simulink model "FOC_physical_2"  (R2024b)
settings: Solver=FixedStepAuto  StartTime=0.0  StopTime=1  FixedStep=1e-6  RelTol=1e-3
undefined symbols (not defined in the file): alpha, DiscIntNeverNeededParam, Down, dspblkCoreblockFVToolHelper, gcbh, GPTRIP1SEL, Ki_current, Ki_q, Ki_s, Ki_speed, Kp_current, Kp_q, Kp_s, Kp_speed, lambda, lamdaM, Ld, Ls, ma, P, Rs, T_max, T_period, TZ1, Up, Vdc
libraries: c2802xlib x7, simulink x7, spsIGBTDiodeLib x6, spsCurrentMeasurementLib x3, eeStairGenerator x2, spsDCVoltageSourceLib x1, spsPermanentMagnetSynchronousMachineLib x1, mcbpositiondecoderlib x1, c281xlib x1, c280xlib x1, spspowerguiLib x1
(part 1 of 2)
settings Model: ExtModeTrigDuration=8  Creator=ahmed  LastModifiedBy=ahmed
settings SolverCC: ZeroCrossAlgorithm=Adaptive
settings OptimizationCC: DefaultParameterBehavior=Inlined  DefaultUnderspecifiedDataType=single  EnhancedBackFolding=on  PassReuseOutputArgsAs=Individual arguments  MaxStackSize=1024  OptimizeBlockOrder=speed  DifferentSizesBufferReuse=on  OptimizationCustomize=off  EfficientTunableParamExpr=on
settings DebuggingCC: IgnoredZcDiagnostic=none  ParameterTunabilityLossMsg=error
settings HardwareCC: ProdBitPerChar=16  ProdBitPerInt=16  ProdBitPerPointer=32  ProdBitPerSizeT=32  ProdBitPerPtrDiffT=32  ProdLargestAtomicInteger=Integer  ProdLargestAtomicFloat=None  ProdWordSize=16  ProdLongLongMode=on  ProdHWDeviceType=Texas Instruments->C2000  HardwareBoardFeatureSet=SoCBlockset
settings SFSimCC: MATLABDynamicMemAlloc=off
settings RTWCC: Description=Embedded Coder  SystemTargetFile=ert.tlc  HardwareBoard=TI Delfino F28379D LaunchPad  TemplateMakefile=ert_default_tmf  Toolchain=Texas Instruments Code Composer Studio (C2000)  CodeProfilingSaveOptions=MetricsOnly
settings CodeAppCC: ForceParamTrailComments=on  IgnoreCustomStorageClasses=off  OperatorAnnotations=on  SimulinkDataObjDesc=on  SFDataObjDesc=on  InsertBlockDesc=on
settings ERTTargetCC: CodeReplacementLibrary=TI C28x  ExtModeTransport=4  ExtModeStaticAlloc=on  ExtModeAutomaticAllocSize=off  ExtModeStaticAllocSize=10000  ExtModeMexFile=ext_xcp  ExtModeIntrfLevel=Level2 - Open

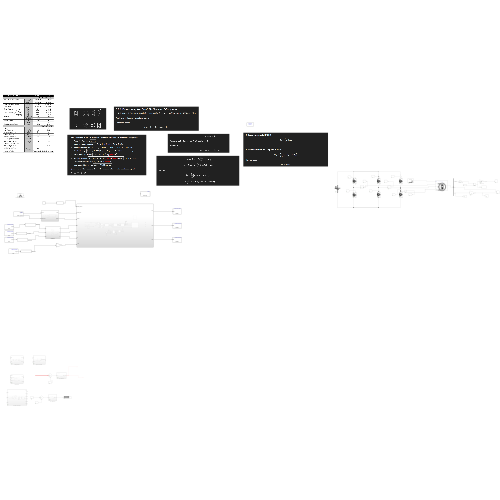
[thumbnail: Simulink's stored preview of the top-level diagram]
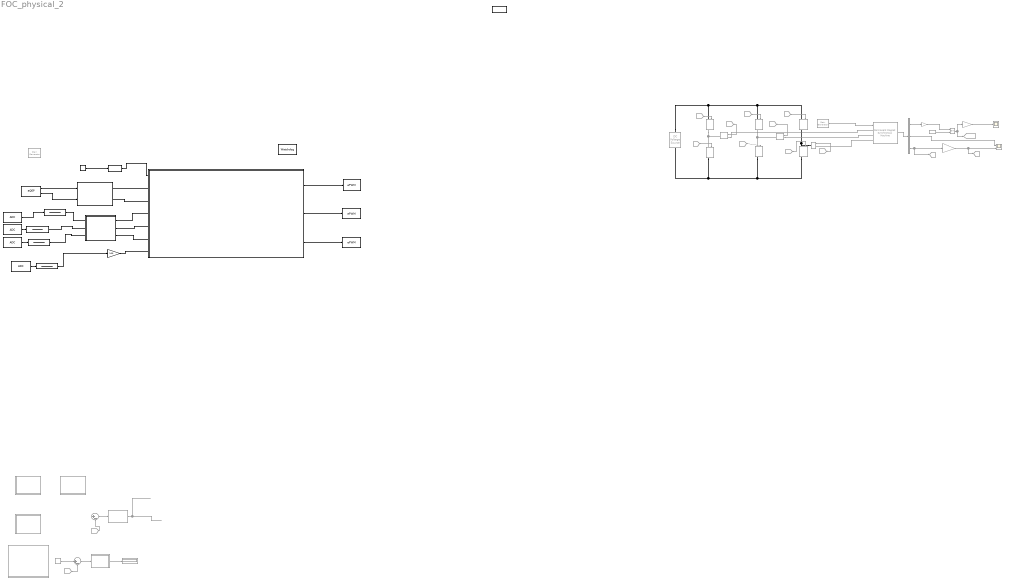
== system FOC_physical_2 ==
  0 to 2pi : Math  Commented=on  Operator=rem
  ADC : c2802xlib/ADC  blkParamProc=C2000_Type4  ADCModule=A  samplingMode=Single sample mode  ADCResolution=12-bit (Single-ended input)  useSOC1=SOC0  useSOC2=SOC0_SOC1  SOCAcquisitionWindow=15  SOCTriggerSource=Software  SOCInterruptTrigger=No ADCINT  Ts=50e-6  dType=uint16  postInterrupt=off  interruptSel=ADCINT1  ADCINTContinuous=on  endma=off  chdma=1  conv1=ADCINA0  conv2=ADCINA0 and ADCINB0  conv1_Type4=ADCIN0  conv2_Type4=ADCIN0 and ADCIN1
      settings: LibrarySourceBlock=c2837xDlib/ADC
  ADC1 : c2802xlib/ADC  blkParamProc=C2000_Type4  ADCModule=A  samplingMode=Single sample mode  ADCResolution=12-bit (Single-ended input)  useSOC1=SOC1  useSOC2=SOC0_SOC1  SOCAcquisitionWindow=15  SOCTriggerSource=ePWM1_ADCSOCA  SOCInterruptTrigger=No ADCINT  Ts=1e-6  dType=uint16  postInterrupt=off  interruptSel=ADCINT1  ADCINTContinuous=on  endma=off  chdma=1  conv1=ADCINA0  conv2=ADCINA0 and ADCINB0  conv1_Type4=ADCIN1  conv2_Type4=ADCIN0 and ADCIN1
      settings: LibrarySourceBlock=c2837xDlib/ADC
  ADC2 : c2802xlib/ADC  blkParamProc=C2000_Type4  ADCModule=A  samplingMode=Single sample mode  ADCResolution=12-bit (Single-ended input)  useSOC1=SOC2  useSOC2=SOC0_SOC1  SOCAcquisitionWindow=15  SOCTriggerSource=ePWM1_ADCSOCA  SOCInterruptTrigger=No ADCINT  Ts=1e-6  dType=uint16  postInterrupt=off  interruptSel=ADCINT1  ADCINTContinuous=on  endma=off  chdma=1  conv1=ADCINA0  conv2=ADCINA0 and ADCINB0  conv1_Type4=ADCIN2  conv2_Type4=ADCIN0 and ADCIN1
      settings: LibrarySourceBlock=c2837xDlib/ADC
  ADC3 : c2802xlib/ADC  blkParamProc=C2000_Type4  ADCModule=A  samplingMode=Single sample mode  ADCResolution=12-bit (Single-ended input)  useSOC1=SOC3  useSOC2=SOC0_SOC1  SOCAcquisitionWindow=15  SOCTriggerSource=ePWM1_ADCSOCA  SOCInterruptTrigger=No ADCINT  Ts=1e-6  dType=uint16  postInterrupt=off  interruptSel=ADCINT1  ADCINTContinuous=on  endma=off  chdma=1  conv1=ADCINA0  conv2=ADCINA0 and ADCINB0  conv1_Type4=ADCIN3  conv2_Type4=ADCIN0 and ADCIN1
      settings: LibrarySourceBlock=c2837xDlib/ADC
  Bus Selector : BusSelector  Commented=on  OutputSignals=theta,Te,w
  "Calibration " : Subsystem
  Cast To Double : DataTypeConversion  OutDataTypeStr=double  SaturateOnIntegerOverflow=off  RndMeth=Floor
  Constant : Constant  Value=1500  OutDataTypeStr=double
  Constant4 : Constant  Commented=on  Value=2*pi
  Current Measurement : spsCurrentMeasurementLib/Current Measurement  Commented=on  PhasorSimulation=off  OutputType=Complex  PSBequivalent=0
  Current Measurement1 : spsCurrentMeasurementLib/Current Measurement  Commented=on  PhasorSimulation=off  OutputType=Complex  PSBequivalent=0
  Current Measurement2 : spsCurrentMeasurementLib/Current Measurement  Commented=on  PhasorSimulation=off  OutputType=Complex  PSBequivalent=0
  DC Voltage Source : spsDCVoltageSourceLib/DC Voltage Source  Commented=on  Amplitude=Vdc  Measurements=None
  "Decoupling " : Subsystem  Commented=on
  Discrete Transfer Fcn{1..3,8} (4 alike) : DiscreteTransferFcn  LoadFcn=dspblkCoreblockFVToolHelper(gcbh,'load');  Numerator=[alpha]  Denominator=[1 (alpha)-1]  RndMeth=Nearest
      settings: CopyFcn=dspblkCoreblockFVToolHelper(gcbh,'copy');  DeleteFcn=dspblkCoreblockFVToolHelper(gcbh,'close');  ModelCloseFcn=dspblkCoreblockFVToolHelper(gcbh,'close');  PreSaveFcn=dspblkCoreblockFVToolHelper(gcbh,'presave');  PostSaveFcn=dspblkCoreblockFVToolHelper(gcbh,'postsave');  CloseFcn=dspblkCoreblockFVToolHelper(gcbh,'close');
  Display5 : Display  Commented=on
  From13 : From  Commented=on  GotoTag=Iq  TagVisibility=global
  From14 : From  Commented=on  GotoTag=Id  TagVisibility=global
  From2 : From  Commented=on  GotoTag=S1  TagVisibility=global
  From3 : From  Commented=on  GotoTag=S3  TagVisibility=global
  From4 : From  Commented=on  GotoTag=S5  TagVisibility=global
  From5 : From  Commented=on  GotoTag=S4  TagVisibility=global
  From6 : From  Commented=on  GotoTag=S6  TagVisibility=global
  From7 : From  Commented=on  GotoTag=S2  TagVisibility=global
  Gain : Gain  Commented=on  Gain=60/(2*pi)
  Gain1 : Gain  Gain=100
  Goto : Goto  Commented=on  GotoTag=N_act
  Goto1 : Goto  Commented=on  GotoTag=theta_rad  TagVisibility=global
  Goto12 : Goto  Commented=on  GotoTag=Ia
  Goto13 : Goto  Commented=on  GotoTag=Ib
  Goto14 : Goto  Commented=on  GotoTag=Ic
  Goto8 : Goto  Commented=on  GotoTag=W_act
  IGBT/Diode{,1..5} (6 alike) : spsIGBTDiodeLib/IGBT//Diode  Commented=on  Ron=1e-3  Rs=1e5  Cs=inf  Measurements=on
  Id : Constant  Commented=on  Value=0
  PI_controller : Subsystem  Commented=on
  PI_controller1 : Subsystem  Commented=on
  Permanent Magnet Synchronous Machine : spsPermanentMagnetSynchronousMachineLib/Permanent Magnet Synchronous Machine  Commented=on  NbPhases=3  FluxDistribution=Sinusoidal  RotorType=Round  MechanicalLoad=Torque Tm  PresetModel=No  ShowDetailedParameters=on  MeasurementBus=on  Resistance=Rs  Inductance=8.5e-3  dqInductances=[6.2e-3 6.2e-3]  La=Ls  MachineConstant=Flux linkage established by magnets (V.s)  Flux=.0620  VoltageCst=44.9822  TorqueCst=0.372  Flat=120  Mechanical=[2.6e-5 9.55e-5 4 .03]  PolePairs=4  InitialConditions=[0,0, 0,0]  InitialConditions5ph=[0 0 0 0 0 0]  RefAngle=Aligned with phase A axis (original Park)  IterativeDiscreteModel=Trapezoidal non iterative  TsBlock=-1  TsPowergui=0
  SPEED_TEST_VALUES : eeStairGenerator/Stair Generator  Commented=on  LabelModeActiveChoice=Discrete  TimeInput=[0.2 .6 1 1.3 1.8 2.2 3]  AmplitudeInput=[200 300 1000 4000 4500 2000 0]  SampleTime=1e-5  RepeatPattern=off
      settings: LibrarySourceBlock=ee_sl_lib/General Control/Stair Generator
  SVPWM Technique : Subsystem  Commented=on
  Scope : Scope  Commented=on
  Scope1 : Scope  Commented=on  NumInputPorts=2
  "Speed Controller " : Subsystem  Commented=on
  Stair Generator2 : eeStairGenerator/Stair Generator  Commented=on  LabelModeActiveChoice=Discrete  TimeInput=[0.3 .7]  AmplitudeInput=[.6 1]  SampleTime=1e-5  RepeatPattern=off  OutDataTypeStr=double
      settings: LibrarySourceBlock=ee_sl_lib/General Control/Stair Generator
  Subsystem : Subsystem
  Subsystem1 : Subsystem
  Sum1 : Sum  Commented=on  Inputs=|+-
  Sum2 : Sum  Commented=on  Inputs=|+-
  Voltage limits : Subsystem  Commented=on
  Watchdog : c281xlib/Watchdog  resetsrc=Input port  sample=-1
      settings: LibrarySourceBlock=c2837xDlib/Watchdog
  ePWM11 : c2802xlib/ePWM  PwmType=C2000_Type4  useModule=ePWM1  ePWMxLINKTBPRD=Not Linked  periodUnits=Clock cycles  timerSource=Specify via dialog  timerPeriod_clk=10000  timerPeriod_sec=0.0001  tbshadow=Counter equals to zero  countingMode=Up-Down  phaseActiveEnable=Disable  phaseDirection=Count down after sync  phaseActive=0  synchronizationEnable=off  dcaevt1Sync=off  dcbevt1Sync=off  synchronizationOption=Counter equals to zero (CTR=Zero)  dcbevt1SyncOut=off  dcaevt1SyncOut=off  cmpdSyncOut=off  cmpcSyncOut=off  cmpbSyncOut=off  zeroSyncOut=off  swfSyncOut=off  perSynchronizationOption=Counter equals to period (CTR=PRD)  clockPrescale=1  HSclockPrescale=1  enswap=off  ePWMxAStatus=on  ePWMxAactionLogic1=Do nothing  ePWMxAactionLogic2=Do nothing  ePWMxAactionLogic3=Clear  ePWMxAactionLogic4=Set  ePWMxAactionLogic5=Do nothing  ePWMxAactionLogic6=Do nothing  ePWMxACSFenable=off  ePWMxACSFvalue=Forcing disable  ePWMxASFreload=Zero  ePWMxBStatus=on  ePWMxBactionLogic1=Do nothing  ePWMxBactionLogic2=Do nothing  ePWMxBactionLogic3=Set  ePWMxBactionLogic4=Clear  ePWMxBactionLogic5=Do nothing  ePWMxBactionLogic6=Do nothing  ePWMxBCSFenable=off  ePWMxBCSFvalue=Forcing disable  ePWMxBSFreload=Zero  ePWNxBOutWay=off  ePWMxLINKCMPA=Not Linked  CMPAUnits=Clock cycles  CMPASource=Input port  CMPAValue_per=0  CMPAValue_clk=0  enCMPAshadow=Counter equals to zero (CTR=Zero)  ePWMxLINKCMPB=Not Linked  CMPBUnits=Clock cycles  CMPBSource=Specify via dialog  CMPBValue_per=50  CMPBValue_clk=32000  enCMPBshadow=Counter equals to zero (CTR=Zero)  ePWMxLINKCMPC=Not Linked  CMPCUnits=Clock cycles  CMPCSource=Specify via dialog  CMPCValue_per=50  CMPCValue_clk=32000  enCMPCshadow=Counter equals to zero (CTR=Zero)  ePWMxLINKCMPD=Not Linked  CMPDUnits=Clock cycles  CMPDSource=Specify via dialog  CMPDValue_per=50  CMPDValue_clk=32000  enCMPDshadow=Counter equals to zero (CTR=Zero)  enableDBePWMxA=on  enableDBePWMxB=on  enhalfcycle=off  DBpolarity=Active high complementary (AHC)  DBedgeDelay=Positive  DBSource_ePWMxA=ePWMxA  DBSource_ePWMxB=ePWMxA  DBPeriodUnits=Clock cycles  DBperiodSource=Specify via dialog  REDperiod=400  FEDperiod=400  REDperiod_sec=0  FEDperiod_sec=0  LoadModeDBRED=Immediate without using shadow  LoadModeDBFED=Immediate without using shadow  adcstartModuleA=on  adcrequestEventA=First event  adcstartEventA=Digital Compare Module A Event 1 start of conversion (DCAEVT1.soc)  adcstartEventA_type2=Counter equals to period (CTR=PRD)  adcstartModuleB=off  adcrequestEventB=First event  adcstartEventB=Counter equals to zero (CTR=Zero)  adcstartEventB_type2=Counter equals to zero (CTR=Zero)  intEn=on  intPrd=First event  intSel=Counter equals to zero (CTR=Zero)  intSel_type2=Counter equals to period (CTR=PRD)  hrpe=off  enHRPWM=off  HRPWM_LoadMode=Counter equals to period (CTR=PRD)  HRPWM_CTLMode=Duty or Period control mode  HRPWM_EDGMode=Both edge  hrpeb=off  enHRPWMB=off  HRPWM_LoadModeB=Counter equals to zero (CTR=ZERO)  HRPWM_CTLModeB=Duty or Period control mode  HRPWM_EDGModeB=Both edge  enHRDBRED=off  enHRDBFED=off  enSFO=on  enautoconv=on  chopperEnable=off  chopperFrequency=1  chopperFirstwidth=1  chopperDuty=12.5%  tripZonesource=Specify via dialog  tzselOSHT1=off  tzselOSHT2=off  tzselOSHT3=off  tzselOSHT4=off  tzselOSHT5=off  tzselOSHT6=off  tzselOSHDCAEV1=off  tzselOSHDCBEV1=off  tzselCBC1=off  tzselCBC2=off  tzselCBC3=off  tzselCBC4=off  tzselCBC5=off  tzselCBC6=off  tzselCBCDCAEV2=off  tzselCBCDCBEV2=off  enTzOstIntr=off  enTzCbcIntr=off  enTzDCAEVT1Intr=off  enTzDCAEVT2Intr=off  enTzDCBEVT1Intr=off  enTzDCBEVT2Intr=off  tzclrCBCLatch=Counter equals to zero (CTR=Zero)  ePWMxAforced=No action  ePWMxBforced=No action  DCAEVT1forced=No action  DCBEVT1forced=No action  DCAEVT2forced=No action  DCBEVT2forced=No action  dcah=Trip Zone 1 input (TZ1)  dcal=Trip Zone 2 input (TZ2)  dcbh=Trip Zone 1 input (TZ1)  dcbl=Trip Zone 2 input (TZ2)  dcah_type2=GPTRIP1SEL/(TZ1)  dcal_type2=GPTRIP1SEL/(TZ1)  dcbh_type2=GPTRIP1SEL/(TZ1)  dcbl_type2=GPTRIP1SEL/(TZ1)  gendcaevt1=Event disabled  gendcaevt2=Event disabled  gendcbevt1=Event disabled  gendcbevt2=Event disabled  dcaevt1src=DCAEVT1 with sync  dcaevt2src=DCAEVT2 with sync  dcbevt1src=DCBEVT1 with sync  dcbevt2src=DCBEVT2 with sync  pulsesel=Counter equals to zero (CTR=Zero)  blankinv=off  blankoffset=0  blankwidth=0  evsrcsel=Filtered version of DCAEVT1 (DCAEVT1FILT)  encape=off
      settings: LibrarySourceBlock=c2837xDlib/ePWM
  ePWM12 : c2802xlib/ePWM  PwmType=C2000_Type4  useModule=ePWM2  ePWMxLINKTBPRD=Not Linked  periodUnits=Clock cycles  timerSource=Specify via dialog  timerPeriod_clk=10000  timerPeriod_sec=0.0001  tbshadow=Counter equals to zero  countingMode=Up-Down  phaseActiveEnable=Disable  phaseDirection=Count down after sync  phaseActive=0  synchronizationEnable=off  dcaevt1Sync=off  dcbevt1Sync=off  synchronizationOption=Disable  dcbevt1SyncOut=off  dcaevt1SyncOut=off  cmpdSyncOut=off  cmpcSyncOut=off  cmpbSyncOut=off  zeroSyncOut=off  swfSyncOut=off  perSynchronizationOption=Counter equals to period (CTR=PRD)  clockPrescale=1  HSclockPrescale=1  enswap=off  ePWMxAStatus=on  ePWMxAactionLogic1=Do nothing  ePWMxAactionLogic2=Do nothing  ePWMxAactionLogic3=Clear  ePWMxAactionLogic4=Set  ePWMxAactionLogic5=Do nothing  ePWMxAactionLogic6=Do nothing  ePWMxACSFenable=off  ePWMxACSFvalue=Forcing disable  ePWMxASFreload=Zero  ePWMxBStatus=on  ePWMxBactionLogic1=Do nothing  ePWMxBactionLogic2=Do nothing  ePWMxBactionLogic3=Set  ePWMxBactionLogic4=Clear  ePWMxBactionLogic5=Do nothing  ePWMxBactionLogic6=Do nothing  ePWMxBCSFenable=off  ePWMxBCSFvalue=Forcing disable  ePWMxBSFreload=Zero  ePWNxBOutWay=off  ePWMxLINKCMPA=Not Linked  CMPAUnits=Clock cycles  CMPASource=Input port  CMPAValue_per=0  CMPAValue_clk=0  enCMPAshadow=Counter equals to zero (CTR=Zero)  ePWMxLINKCMPB=Not Linked  CMPBUnits=Clock cycles  CMPBSource=Specify via dialog  CMPBValue_per=50  CMPBValue_clk=32000  enCMPBshadow=Counter equals to zero (CTR=Zero)  ePWMxLINKCMPC=Not Linked  CMPCUnits=Clock cycles  CMPCSource=Specify via dialog  CMPCValue_per=50  CMPCValue_clk=32000  enCMPCshadow=Counter equals to zero (CTR=Zero)  ePWMxLINKCMPD=Not Linked  CMPDUnits=Clock cycles  CMPDSource=Specify via dialog  CMPDValue_per=50  CMPDValue_clk=32000  enCMPDshadow=Counter equals to zero (CTR=Zero)  enableDBePWMxA=on  enableDBePWMxB=on  enhalfcycle=off  DBpolarity=Active high complementary (AHC)  DBedgeDelay=Positive  DBSource_ePWMxA=ePWMxA  DBSource_ePWMxB=ePWMxA  DBPeriodUnits=Clock cycles  DBperiodSource=Specify via dialog  REDperiod=400  FEDperiod=400  REDperiod_sec=0  FEDperiod_sec=0  LoadModeDBRED=Immediate without using shadow  LoadModeDBFED=Immediate without using shadow  adcstartModuleA=on  adcrequestEventA=First event  adcstartEventA=Digital Compare Module A Event 1 start of conversion (DCAEVT1.soc)  adcstartEventA_type2=Counter equals to period (CTR=PRD)  adcstartModuleB=off  adcrequestEventB=First event  adcstartEventB=Counter equals to zero (CTR=Zero)  adcstartEventB_type2=Counter equals to zero (CTR=Zero)  intEn=on  intPrd=First event  intSel=Counter equals to zero (CTR=Zero)  intSel_type2=Counter equals to period (CTR=PRD)  hrpe=off  enHRPWM=off  HRPWM_LoadMode=Counter equals to period (CTR=PRD)  HRPWM_CTLMode=Duty or Period control mode  HRPWM_EDGMode=Both edge  hrpeb=off  enHRPWMB=off  HRPWM_LoadModeB=Counter equals to zero (CTR=ZERO)  HRPWM_CTLModeB=Duty or Period control mode  HRPWM_EDGModeB=Both edge  enHRDBRED=off  enHRDBFED=off  enSFO=on  enautoconv=on  chopperEnable=off  chopperFrequency=1  chopperFirstwidth=1  chopperDuty=12.5%  tripZonesource=Specify via dialog  tzselOSHT1=off  tzselOSHT2=off  tzselOSHT3=off  tzselOSHT4=off  tzselOSHT5=off  tzselOSHT6=off  tzselOSHDCAEV1=off  tzselOSHDCBEV1=off  tzselCBC1=off  tzselCBC2=off  tzselCBC3=off  tzselCBC4=off  tzselCBC5=off  tzselCBC6=off  tzselCBCDCAEV2=off  tzselCBCDCBEV2=off  enTzOstIntr=off  enTzCbcIntr=off  enTzDCAEVT1Intr=off  enTzDCAEVT2Intr=off  enTzDCBEVT1Intr=off  enTzDCBEVT2Intr=off  tzclrCBCLatch=Counter equals to zero (CTR=Zero)  ePWMxAforced=No action  ePWMxBforced=No action  DCAEVT1forced=No action  DCBEVT1forced=No action  DCAEVT2forced=No action  DCBEVT2forced=No action  dcah=Trip Zone 1 input (TZ1)  dcal=Trip Zone 2 input (TZ2)  dcbh=Trip Zone 1 input (TZ1)  dcbl=Trip Zone 2 input (TZ2)  dcah_type2=GPTRIP1SEL/(TZ1)  dcal_type2=GPTRIP1SEL/(TZ1)  dcbh_type2=GPTRIP1SEL/(TZ1)  dcbl_type2=GPTRIP1SEL/(TZ1)  gendcaevt1=Event disabled  gendcaevt2=Event disabled  gendcbevt1=Event disabled  gendcbevt2=Event disabled  dcaevt1src=DCAEVT1 with sync  dcaevt2src=DCAEVT2 with sync  dcbevt1src=DCBEVT1 with sync  dcbevt2src=DCBEVT2 with sync  pulsesel=Counter equals to zero (CTR=Zero)  blankinv=off  blankoffset=0  blankwidth=0  evsrcsel=Filtered version of DCAEVT1 (DCAEVT1FILT)  encape=off
      settings: LibrarySourceBlock=c2837xDlib/ePWM
  ePWM13 : c2802xlib/ePWM  PwmType=C2000_Type4  useModule=ePWM4  ePWMxLINKTBPRD=Not Linked  periodUnits=Clock cycles  timerSource=Specify via dialog  timerPeriod_clk=10000  timerPeriod_sec=0.0001  tbshadow=Counter equals to zero  countingMode=Up-Down  phaseActiveEnable=Disable  phaseDirection=Count down after sync  phaseActive=0  synchronizationEnable=off  dcaevt1Sync=off  dcbevt1Sync=off  synchronizationOption=Disable  dcbevt1SyncOut=off  dcaevt1SyncOut=off  cmpdSyncOut=off  cmpcSyncOut=off  cmpbSyncOut=off  zeroSyncOut=off  swfSyncOut=off  perSynchronizationOption=Counter equals to period (CTR=PRD)  clockPrescale=1  HSclockPrescale=1  enswap=off  ePWMxAStatus=on  ePWMxAactionLogic1=Do nothing  ePWMxAactionLogic2=Do nothing  ePWMxAactionLogic3=Clear  ePWMxAactionLogic4=Set  ePWMxAactionLogic5=Do nothing  ePWMxAactionLogic6=Do nothing  ePWMxACSFenable=off  ePWMxACSFvalue=Forcing disable  ePWMxASFreload=Zero  ePWMxBStatus=on  ePWMxBactionLogic1=Do nothing  ePWMxBactionLogic2=Do nothing  ePWMxBactionLogic3=Set  ePWMxBactionLogic4=Clear  ePWMxBactionLogic5=Do nothing  ePWMxBactionLogic6=Do nothing  ePWMxBCSFenable=off  ePWMxBCSFvalue=Forcing disable  ePWMxBSFreload=Zero  ePWNxBOutWay=off  ePWMxLINKCMPA=Not Linked  CMPAUnits=Clock cycles  CMPASource=Input port  CMPAValue_per=0  CMPAValue_clk=0  enCMPAshadow=Counter equals to zero (CTR=Zero)  ePWMxLINKCMPB=Not Linked  CMPBUnits=Clock cycles  CMPBSource=Specify via dialog  CMPBValue_per=50  CMPBValue_clk=32000  enCMPBshadow=Counter equals to zero (CTR=Zero)  ePWMxLINKCMPC=Not Linked  CMPCUnits=Clock cycles  CMPCSource=Specify via dialog  CMPCValue_per=50  CMPCValue_clk=32000  enCMPCshadow=Counter equals to zero (CTR=Zero)  ePWMxLINKCMPD=Not Linked  CMPDUnits=Clock cycles  CMPDSource=Specify via dialog  CMPDValue_per=50  CMPDValue_clk=32000  enCMPDshadow=Counter equals to zero (CTR=Zero)  enableDBePWMxA=on  enableDBePWMxB=on  enhalfcycle=off  DBpolarity=Active high complementary (AHC)  DBedgeDelay=Positive  DBSource_ePWMxA=ePWMxA  DBSource_ePWMxB=ePWMxA  DBPeriodUnits=Clock cycles  DBperiodSource=Specify via dialog  REDperiod=400  FEDperiod=400  REDperiod_sec=0  FEDperiod_sec=0  LoadModeDBRED=Immediate without using shadow  LoadModeDBFED=Immediate without using shadow  adcstartModuleA=on  adcrequestEventA=First event  adcstartEventA=Digital Compare Module A Event 1 start of conversion (DCAEVT1.soc)  adcstartEventA_type2=Counter equals to period (CTR=PRD)  adcstartModuleB=off  adcrequestEventB=First event  adcstartEventB=Counter equals to zero (CTR=Zero)  adcstartEventB_type2=Counter equals to zero (CTR=Zero)  intEn=on  intPrd=First event  intSel=Counter equals to zero (CTR=Zero)  intSel_type2=Counter equals to period (CTR=PRD)  hrpe=off  enHRPWM=off  HRPWM_LoadMode=Counter equals to period (CTR=PRD)  HRPWM_CTLMode=Duty or Period control mode  HRPWM_EDGMode=Both edge  hrpeb=off  enHRPWMB=off  HRPWM_LoadModeB=Counter equals to zero (CTR=ZERO)  HRPWM_CTLModeB=Duty or Period control mode  HRPWM_EDGModeB=Both edge  enHRDBRED=off  enHRDBFED=off  enSFO=on  enautoconv=on  chopperEnable=off  chopperFrequency=1  chopperFirstwidth=1  chopperDuty=12.5%  tripZonesource=Specify via dialog  tzselOSHT1=off  tzselOSHT2=off  tzselOSHT3=off  tzselOSHT4=off  tzselOSHT5=off  tzselOSHT6=off  tzselOSHDCAEV1=off  tzselOSHDCBEV1=off  tzselCBC1=off  tzselCBC2=off  tzselCBC3=off  tzselCBC4=off  tzselCBC5=off  tzselCBC6=off  tzselCBCDCAEV2=off  tzselCBCDCBEV2=off  enTzOstIntr=off  enTzCbcIntr=off  enTzDCAEVT1Intr=off  enTzDCAEVT2Intr=off  enTzDCBEVT1Intr=off  enTzDCBEVT2Intr=off  tzclrCBCLatch=Counter equals to zero (CTR=Zero)  ePWMxAforced=No action  ePWMxBforced=No action  DCAEVT1forced=No action  DCBEVT1forced=No action  DCAEVT2forced=No action  DCBEVT2forced=No action  dcah=Trip Zone 1 input (TZ1)  dcal=Trip Zone 2 input (TZ2)  dcbh=Trip Zone 1 input (TZ1)  dcbl=Trip Zone 2 input (TZ2)  dcah_type2=GPTRIP1SEL/(TZ1)  dcal_type2=GPTRIP1SEL/(TZ1)  dcbh_type2=GPTRIP1SEL/(TZ1)  dcbl_type2=GPTRIP1SEL/(TZ1)  gendcaevt1=Event disabled  gendcaevt2=Event disabled  gendcbevt1=Event disabled  gendcbevt2=Event disabled  dcaevt1src=DCAEVT1 with sync  dcaevt2src=DCAEVT2 with sync  dcbevt1src=DCBEVT1 with sync  dcbevt2src=DCBEVT2 with sync  pulsesel=Counter equals to zero (CTR=Zero)  blankinv=off  blankoffset=0  blankwidth=0  evsrcsel=Filtered version of DCAEVT1 (DCAEVT1FILT)  encape=off
      settings: LibrarySourceBlock=c2837xDlib/ePWM
  eQEP : c280xlib/eQEP  useModule=eQEP1  pcInputmode=Quadrature-count  externalClockrate=2x resolution: Count the rising/falling edge  swapPolarityselection=Clockwise  qdfOutputport=off  qapPolarityselection=off  qbpPolarityselection=off  qipPolarityselection=off  qspPolarityselection=off  igatePolarityselection=off  sampleTime=0.0001  pcOutputport=on  pcMaximumvalue=4*2000  indexInitializationcheck=off  indexInitializationevent=Rising edge  strobeInitializationcheck=off  strobeInitializationevent=Rising edge  softwareInitializationcheck=off  softwareInitializationsource=Set to init value at start up  softwareInitializationmode=on  pcInitialvalue=2147483648  pcResetmode=Reset on the maximum position  ieloutputport=on  indexEventlatch=Rising edge  seloutputport=off  strobeEventlatch=Rising edge  pcefOutputport=off  enableEqepcapture=on  qctmrOutputport=off  qcprdOutputport=off  captureTimerprescaler=128  upEventprescaler=128  overflowErrorflag=off  directionErrorflag=off  captureTimerposition=On position counter read  unitTimerperiod=100000000  captureTimerlatch=off  capturePeriodlatch=off  positionCounterlatch=off  soenPolarityselection=off  spselPolarityselection=Index pin is used for sync output  compareValuesource=Specify via dialog  shadowMode=Load on QPOSCNT=0  compareValue=4294967295  syncOutputwidth=1  polaritySyncoutput=Active high  watchdogEnable=off  watchdogTimer=65535  outport1Datatype=auto  outport2Datatype=auto  outport3Datatype=auto  outport4Datatype=auto  outport5Datatype=auto  outport6Datatype=auto  outport7Datatype=auto  outport8Datatype=auto  outport9Datatype=auto  outport10Datatype=auto  outport11Datatype=auto  outport12Datatype=auto  eqepinterrupt_pce=off  eqepinterrupt_qpe=off  eqepinterrupt_qdc=off  eqepinterrupt_wto=off  eqepinterrupt_pcu=off  eqepinterrupt_pco=off  eqepinterrupt_pcr=off  eqepinterrupt_pcm=off  eqepinterrupt_sel=off  eqepinterrupt_iel=off  eqepinterrupt_uto=off  pheOutputport=off  watchdogOutputport=off  outport13Datatype=auto  outport14Datatype=auto
      settings: LibrarySourceBlock=c2837xDlib/eQEP
  mech to elec : Gain  Commented=on  Gain=P
  powergui : spspowerguiLib/powergui  Priority=1  SimulationMode=Discrete  SampleTime=1e-5  frequency=60  Iterations=50  frequencyindice=0  Pbase=100e6  ErrMax=1e-4  UnitsV=kV  UnitsW=MW  buscounter=0  FunctionMessages=off  echomessages=off  EnableUseOfTLC=off  CurrentSourceSwitches=off  DisableSnubberDevices=off  DisableRonSwitches=off  DisableVfSwitches=off  DisplayEquations=off  AutomaticDiscreteSolvers=off  SolverType=Tustin/Backward Euler (TBE)  Interpol=off  ExternalGateDelay=off  methode=off  Ts=100  x0status=blocks  SPID=on  SwTol=0  HookPort=off  NonlinearTolerance=1e-4  nMaxIteration=100  ContinueOnMaxIteration=off  RestoreLinks=warning  ResistiveCurrentMeasurement=off  Frange=[0:2:500]  Ylog=off  Xlog=on  ShowGrid=off  save=off  variable=ZData  structure=0  ZoomFFT=off  StartTime=0.0  cycles=1  DisplayStyle=1  fundamental=60  FreqAxis=off  MaxFrequency=1000  frequencyindicesteady=1  RmsSteady=1  display=off
  rad to deg : Gain  Commented=on  Gain=180/pi
  wires:
  Permanent Magnet Synchronous Machine/1 -> Bus Selector/1
  From3/1 -> IGBT/Diode1/1
  From6/1 -> IGBT/Diode3/1
  From4/1 -> IGBT/Diode4/1
  From5/1 -> IGBT/Diode2/1
  From2/1 -> IGBT/Diode/1
  From7/1 -> IGBT/Diode5/1
  PI_controller1/1(Vd_hat) -> Display5/1
  Id/1 -> Sum1/1
  From14/1 -> Sum1/2
  Current Measurement/1 -> Goto12/1
  Current Measurement1/1 -> Goto13/1
  Sum1/1 -> PI_controller1/1(e_d)
  ? -> Sum2/1
  Sum2/1 -> PI_controller/1(e_q)
  PI_controller/1(Vq_hat) -> ?
  From13/1 -> Sum2/2
  Bus Selector/2 -> Scope1/1  "<Te>"
  Bus Selector/3 -> Goto8/1, Gain/1  "<w>"
  Bus Selector/1 -> mech to elec/1  "<theta>"
  0 to 2pi/1 -> rad to deg/1, Goto1/1
  Constant4/1 -> 0 to 2pi/2
  rad to deg/1 -> Scope/1  "degrees"
  mech to elec/1 -> 0 to 2pi/1
  Gain/1 -> Goto/1, Scope1/2
  Current Measurement2/1 -> Goto14/1
  Stair Generator2/1 -> Permanent Magnet Synchronous Machine/1
  Subsystem/1(TS1) -> ePWM11/1
  Subsystem/2(TS3) -> ePWM12/1
  Subsystem/3(TS5) -> ePWM13/1
  eQEP/1 -> Subsystem1/1(Count)
  eQEP/2 -> Subsystem1/2(IndexCount)
  Subsystem1/1(theta) -> Subsystem/2(Theata_elec)
  Subsystem1/2(Speed) -> Subsystem/3(Speed)
  ADC/1 -> Discrete Transfer Fcn8/1
  ADC1/1 -> Discrete Transfer Fcn1/1
  ADC2/1 -> Discrete Transfer Fcn2/1
  "Calibration "/1(Out1) -> Subsystem/4(Iu)
  "Calibration "/2(Out2) -> Subsystem/5(Iv)
  "Calibration "/3(Out3) -> Subsystem/6(Iw)
  ADC3/1 -> Discrete Transfer Fcn3/1
  Gain1/1 -> Subsystem/7(V_DC)
  Constant/1 -> Cast To Double/1
  Cast To Double/1 -> Subsystem/1(SPEED_INPUT)
  Discrete Transfer Fcn8/1 -> "Calibration "/1(In1)  "Discrete TF"
  Discrete Transfer Fcn1/1 -> "Calibration "/2(In2)  "Discrete TF"
  Discrete Transfer Fcn2/1 -> "Calibration "/3(In3)  "Discrete TF"
  Discrete Transfer Fcn3/1 -> Gain1/1  "Discrete TF"
  connections:
  DC Voltage Source/RConn1 -- IGBT/Diode4/LConn1 -- IGBT/Diode1/LConn1 -- IGBT/Diode/LConn1
  Current Measurement/LConn1 -- IGBT/Diode/RConn1 -- IGBT/Diode2/LConn1
  Current Measurement2/LConn1 -- IGBT/Diode4/RConn1 -- IGBT/Diode5/LConn1
  DC Voltage Source/LConn1 -- IGBT/Diode5/RConn1 -- IGBT/Diode3/RConn1 -- IGBT/Diode2/RConn1
  Current Measurement1/LConn1 -- IGBT/Diode1/RConn1 -- IGBT/Diode3/LConn1
  Current Measurement/RConn1 -- Permanent Magnet Synchronous Machine/LConn1
  Current Measurement1/RConn1 -- Permanent Magnet Synchronous Machine/LConn2
  Permanent Magnet Synchronous Machine/LConn3 -- Current Measurement2/RConn1

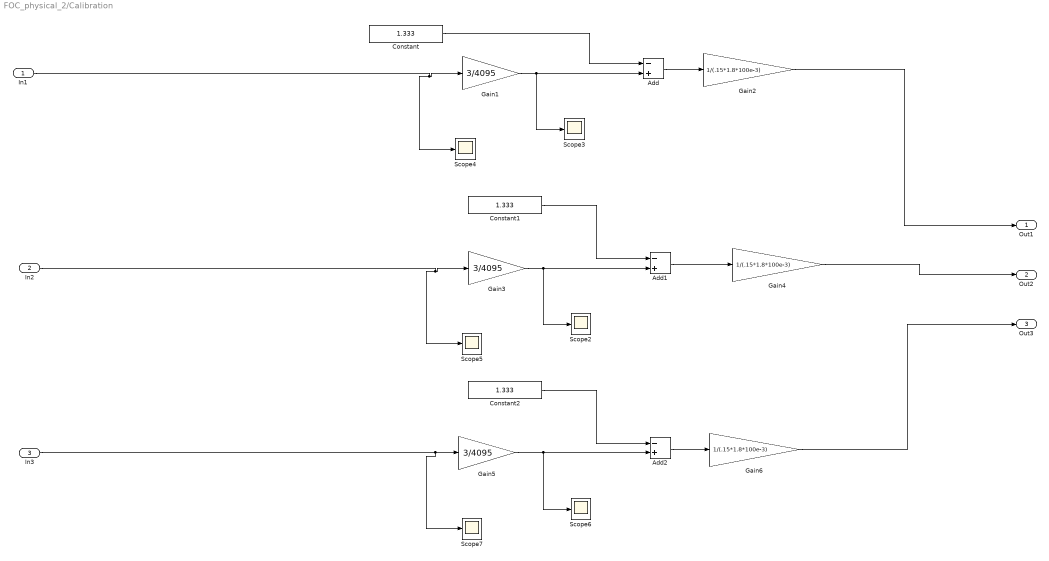
== system FOC_physical_2/Calibration  ==
  In1 : Inport
  In2 : Inport  Port=2
  In3 : Inport  Port=3
  Add : Sum  Inputs=-+
  Add1 : Sum  Inputs=-+
  Add2 : Sum  Inputs=-+
  Constant : Constant  Value=1.333
  Constant1 : Constant  Value=1.333
  Constant2 : Constant  Value=1.333
  Gain1 : Gain  Gain=3/4095
  Gain2 : Gain  Gain=1/(.15*1.8*100e-3)
  Gain3 : Gain  Gain=3/4095
  Gain4 : Gain  Gain=1/(.15*1.8*100e-3)
  Gain5 : Gain  Gain=3/4095
  Gain6 : Gain  Gain=1/(.15*1.8*100e-3)
  Scope{2..7} (6 alike) : Scope
  Out1 : Outport
  Out2 : Outport  Port=2
  Out3 : Outport  Port=3
  wires:
  Gain3/1 -> Add1/2, Scope2/1
  In3/1 -> Scope7/1, Gain5/1
  Gain1/1 -> Scope3/1, Add/2
  In1/1 -> Scope4/1, Gain1/1
  Gain5/1 -> Scope6/1, Add2/2
  Add2/1 -> Gain6/1
  Gain2/1 -> Out1/1
  In2/1 -> Gain3/1, Scope5/1
  Constant1/1 -> Add1/1
  Constant/1 -> Add/1
  Add/1 -> Gain2/1
  Add1/1 -> Gain4/1
  Constant2/1 -> Add2/1
  Gain6/1 -> Out3/1
  Gain4/1 -> Out2/1

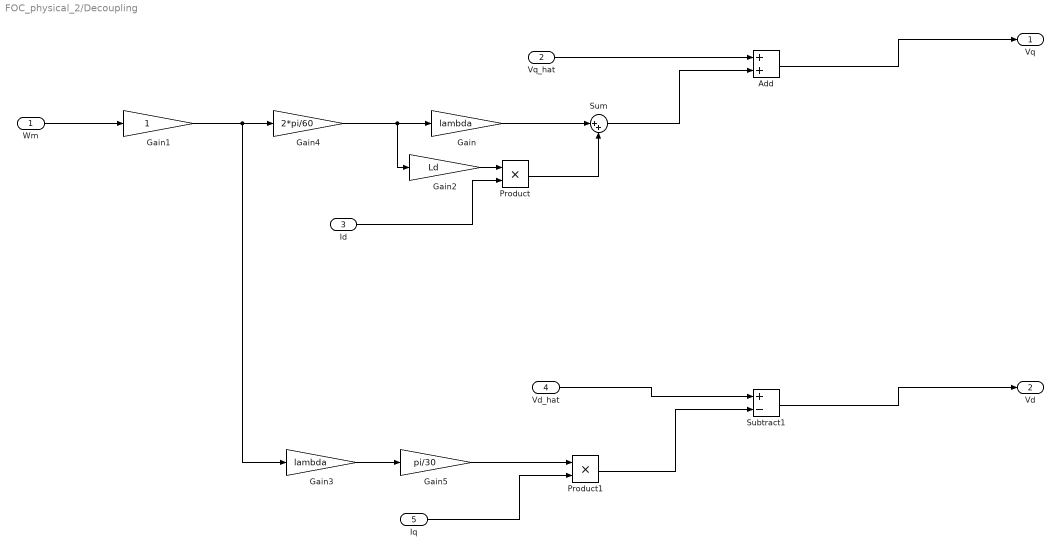
== system FOC_physical_2/Decoupling  ==
  Wm : Inport
  Vq_hat : Inport  Port=2
  Id : Inport  Port=3
  Vd_hat : Inport  Port=4
  Iq : Inport  Port=5
  Add : Sum
  Gain : Gain  Gain=lambda
  Gain1 : Gain
  Gain2 : Gain  Gain=Ld
  Gain3 : Gain  Gain=lambda
  Gain4 : Gain  Gain=2*pi/60
  Gain5 : Gain  Gain=pi/30
  Product : Product
  Product1 : Product
  Subtract1 : Sum  Inputs=+-
  Sum : Sum  Inputs=|++
  Vq : Outport
  Vd : Outport  Port=2
  wires:
  Vq_hat/1 -> Add/1
  Vd_hat/1 -> Subtract1/1
  Wm/1 -> Gain1/1
  Gain1/1 -> Gain4/1, Gain3/1
  Gain2/1 -> Product/1
  Id/1 -> Product/2
  Product/1 -> Sum/2
  Gain/1 -> Sum/1
  Sum/1 -> Add/2
  Gain3/1 -> Gain5/1
  Product1/1 -> Subtract1/2
  Iq/1 -> Product1/2
  Gain4/1 -> Gain2/1, Gain/1
  Add/1 -> Vq/1
  Subtract1/1 -> Vd/1
  Gain5/1 -> Product1/1

== system FOC_physical_2/PI_controller ==
  note: Kp = ((2*zeta*wn)-(Rs/ld))*Ld
  note: Kp = (Wn^2)*Ld
  e_q : Inport
  Add : Sum
  Display : Display
  Integrator : Integrator
  Ki : Gain  Gain=Ki_q
  Kp : Gain  Gain=Kp_q
  Product : Product
  Scope : Scope
  Vq_hat : Outport
  wires:
  Kp/1 -> Add/1
  Add/1 -> Vq_hat/1, Display/1
  e_q/1 -> Ki/1, Kp/1
  [Stop_q_integrator] -> Scope/1, Product/2
  Product/1 -> Integrator/1
  Integrator/1 -> Add/2
  Ki/1 -> Product/1

== system FOC_physical_2/PI_controller1 ==
  e_d : Inport
  Integrator : Integrator
  Ki : Gain  Gain=Ki_q
  Kp : Gain  Gain=Kp_q
  Product : Product
  Sum : Sum  Inputs=|++
  Time Scope : Scope
  Vd_hat : Outport
  wires:
  Kp/1 -> Sum/1
  e_d/1 -> Ki/1, Kp/1
  Sum/1 -> Vd_hat/1
  Product/1 -> Integrator/1
  [Stop_d_integrator] -> Product/2, Time Scope/1
  Integrator/1 -> Sum/2
  Ki/1 -> Product/1

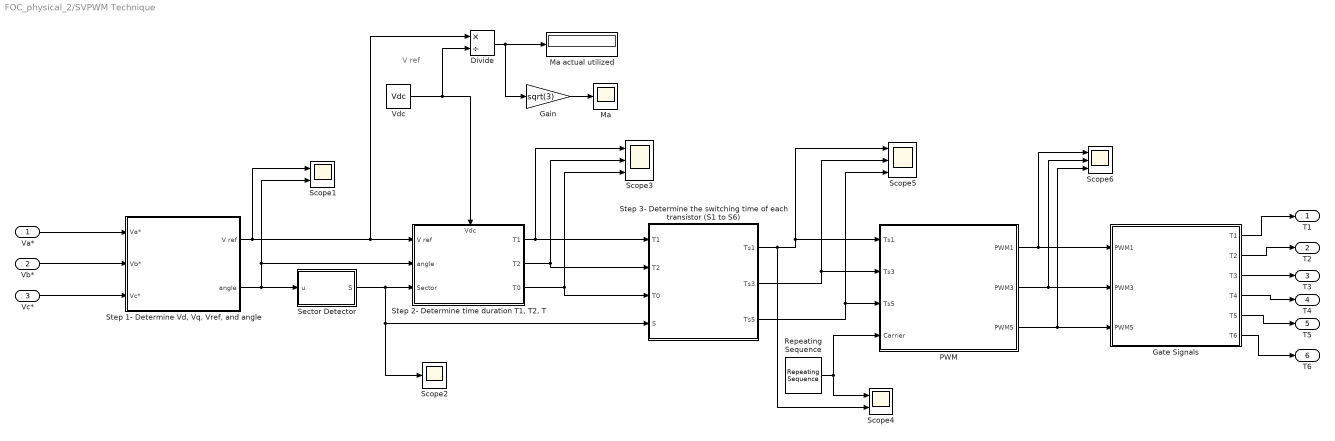
== system FOC_physical_2/SVPWM Technique ==
  note: V ref
  Va* : Inport
  Vb* : Inport  Port=2
  Vc* : Inport  Port=3
  Divide : Product  Inputs=*/
  Gain : Gain  Gain=sqrt(3)
  Gate Signals : Subsystem
  Ma : Scope
  Ma actual utilized : Display
  PWM : Subsystem
  Repeating Sequence : simulink/Sources/Repeating Sequence  rep_seq_t=[ 0 (T_period)/2 (T_period) ]  rep_seq_y=[ 0 (T_period) 0 ]
  Scope1 : Scope  NumInputPorts=2
  Scope2 : Scope
  Scope3 : Scope  NumInputPorts=3
  Scope4 : Scope  NumInputPorts=2
  Scope5 : Scope  NumInputPorts=3
  Scope6 : Scope  NumInputPorts=3
  Sector Detector : MATLAB Function  TreatAsAtomicUnit=on
  "Step 1- Determine Vd, Vq, Vref, and angle" : Subsystem
  "Step 2- Determine time duration T1, T2, T" : Subsystem
      settings: PortSchema="{\"entries\":[{\"content\":{\"sides\":[{\"content\":{\"connectorIds\":[\"In1\",\"In2\",\"In3\"]},\"type\":\"ConnectorPlacement.EquallySpacedRectSide\",\"uuid\":\"2dad9b71-fb55-40e3-9250-08671b06fd76\"},{\"content\":{\"connectorIds\":[\"Out1\",\"Out2\",\"Out3\"],\"side\":\"RIGHT\"},\"type\":\"ConnectorPlacement.EquallySpacedRectSide\",\"uuid\":\"fd9577f6-2035-4946-b366-efd909fd578d\"},{\"content\":{\"connectorIds\":[\"In4\"],\"side\":\"TOP\"},\"type\":\"ConnectorPlacement.EquallySpacedRectSide\",\"uuid\":\"03f93542-188d-4be0-9359-187a882052ac\"}]},\"type\":\"ConnectorPlacement.EquallySpacedConnector\",\"uuid\":\"0cec5607-3333-48e6-b527-ee7f13af7673\"}],\"packageUris\":[\"http://schema.mathworks.com/mf0/Connector/R2020b\"],\"version\":\"1.0\"}"
  "Step 3- Determine the switching time of each transistor (S1 to S6) " : Subsystem
  Vdc : Constant  Value=Vdc
  T1 : Outport
  T2 : Outport  Port=2
  T3 : Outport  Port=3
  T4 : Outport  Port=4
  T5 : Outport  Port=5
  T6 : Outport  Port=6
  wires:
  Vc*/1 -> "Step 1- Determine Vd, Vq, Vref, and angle"/3(Vc*)
  Vb*/1 -> "Step 1- Determine Vd, Vq, Vref, and angle"/2(Vb*)
  "Step 1- Determine Vd, Vq, Vref, and angle"/1(V ref) -> "Step 2- Determine time duration T1, T2, T"/1(V ref), Divide/1, Scope1/1
  Gate Signals/3(T3) -> T3/1
  Gate Signals/1(T1) -> T1/1
  Gate Signals/5(T5) -> T5/1
  "Step 3- Determine the switching time of each transistor (S1 to S6) "/3(Ts5) -> PWM/3(Ts5), Scope5/3
  "Step 3- Determine the switching time of each transistor (S1 to S6) "/2(Ts3) -> PWM/2(Ts3), Scope5/2
  "Step 3- Determine the switching time of each transistor (S1 to S6) "/1(Ts1) -> Scope4/2, PWM/1(Ts1), Scope5/1
  Gate Signals/6(T6) -> T6/1
  PWM/3(PWM5) -> Gate Signals/3(PWM5), Scope6/3
  Divide/1 -> Gain/1, Ma actual utilized/1
  Va*/1 -> "Step 1- Determine Vd, Vq, Vref, and angle"/1(Va*)
  "Step 2- Determine time duration T1, T2, T"/2(T2) -> "Step 3- Determine the switching time of each transistor (S1 to S6) "/2(T2), Scope3/2
  PWM/1(PWM1) -> Gate Signals/1(PWM1), Scope6/1
  "Step 2- Determine time duration T1, T2, T"/1(T1) -> "Step 3- Determine the switching time of each transistor (S1 to S6) "/1(T1), Scope3/1
  Gate Signals/2(T2) -> T2/1
  Vdc/1 -> "Step 2- Determine time duration T1, T2, T"/4(Vdc), Divide/2
  Sector Detector/1(S) -> Scope2/1, "Step 3- Determine the switching time of each transistor (S1 to S6) "/4(S), "Step 2- Determine time duration T1, T2, T"/3(Sector)
  Gate Signals/4(T4) -> T4/1
  PWM/2(PWM3) -> Gate Signals/2(PWM3), Scope6/2
  "Step 1- Determine Vd, Vq, Vref, and angle"/2(angle) -> Sector Detector/1(u), "Step 2- Determine time duration T1, T2, T"/2(angle), Scope1/2
  "Step 2- Determine time duration T1, T2, T"/3(T0) -> "Step 3- Determine the switching time of each transistor (S1 to S6) "/3(T0), Scope3/3
  Repeating Sequence/1 -> PWM/4(Carrier), Scope4/1
  Gain/1 -> Ma/1

== system FOC_physical_2/Speed Controller  ==
  In1 : Inport
  Wm : Inport  Port=2
  Abs : Abs  SaturateOnIntegerOverflow=off
  Abs1 : Abs  SaturateOnIntegerOverflow=off
  Add : Sum
  Compare To Constant : simulink/Logic and Bit Operations/Compare To Constant  relop=<=  const=.0001  OutDataTypeStr=boolean
  Display1 : Display
  Gain : Gain  Gain=Kp_s
  Gain1 : Gain  Gain=Ki_s
  Gain2 : Gain  Gain=2*pi/60
  Integrator : Integrator  ExternalReset=falling
  Product : Product  Inputs=3
  Relay : Relay  OnSwitchValue=100  OffSwitchValue=-100
  Saturation : Saturate  UpperLimit=11  LowerLimit=-11
  Sum : Sum  Inputs=|-+
  Sum1 : Sum  Inputs=|+-
  Iq command : Outport
  wires:
  Gain/1 -> Add/1
  Add/1 -> Saturation/1, Sum/2
  Gain2/1 -> Gain/1, Gain1/1
  In1/1 -> Sum1/1  "Wm"
  Wm/1 -> Abs/1, Sum1/2
  Sum1/1 -> Gain2/1
  Abs/1 -> Relay/1
  Product/1 -> Integrator/1
  Saturation/1 -> Sum/1, Iq command/1, Display1/1
  Abs1/1 -> Compare To Constant/1
  Sum/1 -> Abs1/1
  Compare To Constant/1 -> Product/1
  Gain1/1 -> Product/2
  Relay/1 -> Integrator/2, Product/3
  Integrator/1 -> Add/2

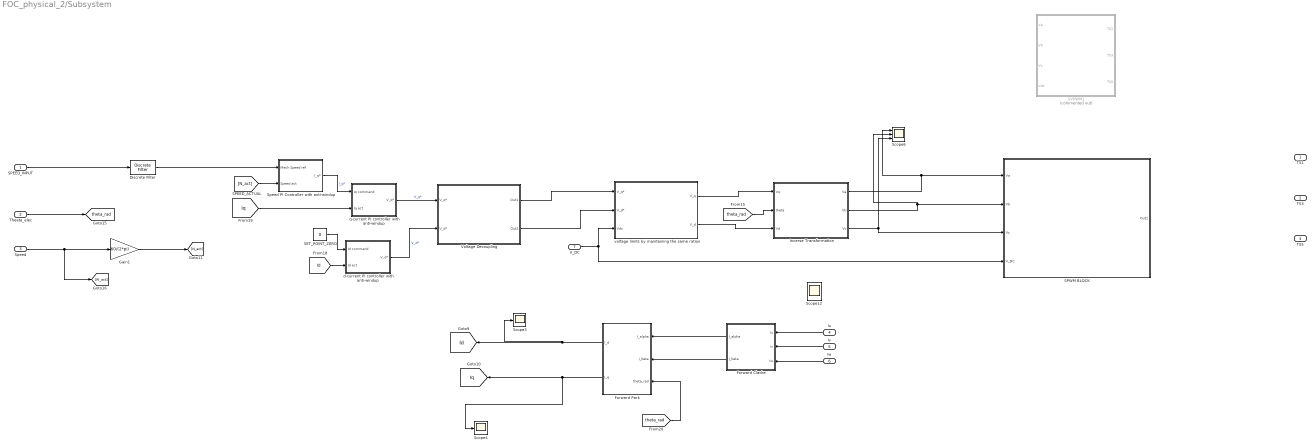
== system FOC_physical_2/Subsystem ==
  SPEED_INPUT : Inport
  Theata_elec : Inport  Port=2
  Speed : Inport  Port=3
  Iu : Inport  Port=4
  Iv : Inport  Port=5
  Iw : Inport  Port=6
  V_DC : Inport  Port=7
  Discrete Filter : DiscreteFilter
  Forward Clacke : Subsystem
  Forward Park : Subsystem
  Gain1 : Gain  Gain=60/(2*pi)
  Inverse Transformation : Subsystem
  SET_POINT_ZERO : Constant  Value=0
  SPWM BLOCK : Subsystem
  SVPWM1 : Subsystem  Commented=on
  Scope12 : Scope  NumInputPorts=3
  Scope3 : Scope
  Scope4 : Scope
  Scope6 : Scope  NumInputPorts=3
  Speed PI Controller with anti-windup : Subsystem
  "Voltage Decoupling " : Subsystem
  d-current PI controller with anti-windup : Subsystem
  q-current PI controller with anti-windup : Subsystem
  voltage limits by maintaining the same ration : Subsystem
  TS1 : Outport
  TS3 : Outport  Port=2
  TS5 : Outport  Port=3
  tag scope: Id=global, Iq=global, theta_rad=global
  wires:
  Inverse Transformation/2(Vb) -> Scope6/2, SPWM BLOCK/2(Vb)
  [Id] -> d-current PI controller with anti-windup/2(Id act)
  Inverse Transformation/1(Va) -> Scope6/1, SPWM BLOCK/1(Va)
  [N_act] -> Speed PI Controller with anti-windup/2(Speed act)
  Inverse Transformation/3(Vc) -> Scope6/3, SPWM BLOCK/3(Vc)
  Speed PI Controller with anti-windup/1(I_q*) -> q-current PI controller with anti-windup/1(Iq command)  "I_q*"
  Forward Clacke/2(I_beta) -> Forward Park/2(I_beta)
  Forward Clacke/1(I_alpha) -> Forward Park/1(I_alpha)
  SET_POINT_ZERO/1 -> d-current PI controller with anti-windup/1(Id command)
  Discrete Filter/1 -> Speed PI Controller with anti-windup/1(Mech Speed ref)
  Forward Park/2(I_q) -> [Iq], Scope4/1
  [theta_rad] -> Inverse Transformation/2(theta)
  voltage limits by maintaining the same ration/2(V_d) -> Inverse Transformation/3(Vd)
  [theta_rad] -> Forward Park/3(theta_rad)
  Forward Park/1(I_d) -> [Id], Scope3/1
  SPEED_INPUT/1 -> Discrete Filter/1
  "Voltage Decoupling "/2(Out2) -> voltage limits by maintaining the same ration/2(V_d*)
  d-current PI controller with anti-windup/1(V_d*) -> "Voltage Decoupling "/2(V_d*)  "V_d*"
  "Voltage Decoupling "/1(Out1) -> voltage limits by maintaining the same ration/1(V_q*)
  q-current PI controller with anti-windup/1(V_q*) -> "Voltage Decoupling "/1(V_q*)  "V_q*"
  [Iq] -> q-current PI controller with anti-windup/2(Iq act)
  voltage limits by maintaining the same ration/1(V_q) -> Inverse Transformation/1(Vq)
  Speed/1 -> [W_act], Gain1/1
  Gain1/1 -> [N_act]
  Theata_elec/1 -> [theta_rad]
  Iu/1 -> Forward Clacke/1(Iu)
  Iv/1 -> Forward Clacke/2(Iv)
  Iw/1 -> Forward Clacke/3(Iw)
  V_DC/1 -> SPWM BLOCK/4(V_DC), voltage limits by maintaining the same ration/3(Vdc)

== system FOC_physical_2/Subsystem1 ==
  Count : Inport
  IndexCount : Inport  Port=2
  Cast To Double : DataTypeConversion  OutDataTypeStr=double  SaturateOnIntegerOverflow=off  RndMeth=Floor
  Constant4 : Constant  Value=1/10000
  Discrete Transfer Fcn8 : DiscreteTransferFcn  LoadFcn=dspblkCoreblockFVToolHelper(gcbh,'load');  Numerator=[alpha]  Denominator=[1 (alpha)-1]  RndMeth=Nearest
      settings: CopyFcn=dspblkCoreblockFVToolHelper(gcbh,'copy');  DeleteFcn=dspblkCoreblockFVToolHelper(gcbh,'close');  ModelCloseFcn=dspblkCoreblockFVToolHelper(gcbh,'close');  PreSaveFcn=dspblkCoreblockFVToolHelper(gcbh,'presave');  PostSaveFcn=dspblkCoreblockFVToolHelper(gcbh,'postsave');  CloseFcn=dspblkCoreblockFVToolHelper(gcbh,'close');
  MATLAB Function : MATLAB Function  TreatAsAtomicUnit=on
  Quadrature Decoder : mcbpositiondecoderlib/Quadrature Decoder  EncoderSlitsPerRevolution=2000  EncoderCountsPerSlit=4  CounterSize=16 bits  ExternalIndexCount=on  PositionUnit=Radians  PositionDataType=single  ParameterInputType=off  CountsPerRevInverseDataType=single
      settings: LibrarySourceBlock=mcbhdllib/Sensor Decoders/Quadrature Decoder
  mech to elec2 : Gain  Gain=60/(2*pi)  OutDataTypeStr=double
  theta : Outport
  Speed : Outport  Port=2
  wires:
  IndexCount/1 -> Quadrature Decoder/2
  Quadrature Decoder/1 -> Cast To Double/1
  Count/1 -> Quadrature Decoder/1
  MATLAB Function/1(speed_rad_s) -> mech to elec2/1
  mech to elec2/1 -> Discrete Transfer Fcn8/1
  Cast To Double/1 -> MATLAB Function/1(theta), theta/1
  Constant4/1 -> MATLAB Function/2(Ts)
  Discrete Transfer Fcn8/1 -> Speed/1  "Discrete TF"

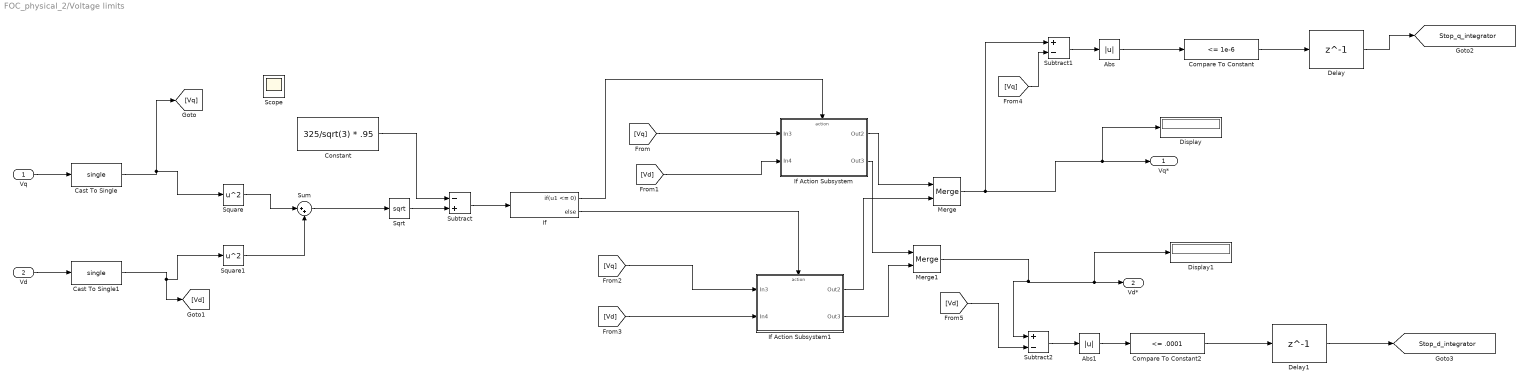
== system FOC_physical_2/Voltage limits ==
  Vq : Inport
  Vd : Inport  Port=2
  Abs : Abs  SaturateOnIntegerOverflow=off
  Abs1 : Abs  SaturateOnIntegerOverflow=off
  Cast To Single : DataTypeConversion  OutDataTypeStr=single  SaturateOnIntegerOverflow=off  RndMeth=Floor
  Cast To Single1 : DataTypeConversion  OutDataTypeStr=single  SaturateOnIntegerOverflow=off  RndMeth=Floor
  Compare To Constant : simulink/Logic and Bit Operations/Compare To Constant  relop=<=  const=1e-6  OutDataTypeStr=boolean
  Compare To Constant2 : simulink/Logic and Bit Operations/Compare To Constant  relop=<=  const=.0001  OutDataTypeStr=boolean
  Constant : Constant  Value=325/sqrt(3) * .95
  Delay : Delay  DelayLength=1
  Delay1 : Delay  DelayLength=1
  Display : Display
  Display1 : Display
  If : If  IfExpression=u1 <= 0
  If Action Subsystem : Subsystem  TreatAsAtomicUnit=on
  If Action Subsystem1 : Subsystem  TreatAsAtomicUnit=on
  Merge : Merge
  Merge1 : Merge
  Scope : Scope
  Sqrt : Sqrt
  Square : Math  Operator=square
  Square1 : Math  Operator=square
  Subtract : Sum  Inputs=-+
  Subtract1 : Sum  Inputs=+-
  Subtract2 : Sum  Inputs=+-
  Sum : Sum  Inputs=|++
  Vq* : Outport
  Vd* : Outport  Port=2
  tag scope: Stop_d_integrator=global, Stop_q_integrator=global
  wires:
  Vq/1 -> Cast To Single/1
  Vd/1 -> Cast To Single1/1
  Square/1 -> Sum/1
  Square1/1 -> Sum/2
  Sum/1 -> Sqrt/1
  Sqrt/1 -> Subtract/2
  Constant/1 -> Subtract/1
  Subtract/1 -> If/1
  If/1 -> If Action Subsystem/Action
  If/2 -> If Action Subsystem1/Action
  [Vq] -> If Action Subsystem/1(In3)
  [Vd] -> If Action Subsystem/2(In4)
  [Vq] -> If Action Subsystem1/1(In3)
  [Vd] -> If Action Subsystem1/2(In4)
  If Action Subsystem/1(Out2) -> Merge/1
  If Action Subsystem1/1(Out2) -> Merge/2
  If Action Subsystem/2(Out3) -> Merge1/1
  If Action Subsystem1/2(Out3) -> Merge1/2
  Merge/1 -> Subtract1/1, Display/1, Vq*/1
  Subtract1/1 -> Abs/1
  Abs/1 -> Compare To Constant/1
  Abs1/1 -> Compare To Constant2/1
  Subtract2/1 -> Abs1/1
  [Vd] -> Subtract2/2
  Compare To Constant/1 -> Delay/1
  Compare To Constant2/1 -> Delay1/1
  Delay/1 -> [Stop_q_integrator]
  Delay1/1 -> [Stop_d_integrator]
  Merge1/1 -> Subtract2/1, Display1/1, Vd*/1
  Cast To Single/1 -> [Vq], Square/1
  Cast To Single1/1 -> [Vd], Square1/1
  [Vq] -> Subtract1/2

== system FOC_physical_2/SVPWM Technique/Gate Signals ==
  PWM1 : Inport
  PWM3 : Inport  Port=2
  PWM5 : Inport  Port=3
  NOT : Logic  Operator=NOT  IconShape=distinctive  AllPortsSameDT=off  OutDataTypeStr=boolean
  NOT1 : Logic  Operator=NOT  IconShape=distinctive  AllPortsSameDT=off  OutDataTypeStr=boolean
  NOT2 : Logic  Operator=NOT  IconShape=distinctive  AllPortsSameDT=off  OutDataTypeStr=boolean
  T1 : Outport
  T2 : Outport  Port=2
  T3 : Outport  Port=3
  T4 : Outport  Port=4
  T5 : Outport  Port=5
  T6 : Outport  Port=6
  wires:
  NOT2/1 -> T2/1
  PWM5/1 -> NOT2/1, T5/1
  PWM3/1 -> NOT1/1, T3/1
  NOT1/1 -> T6/1
  NOT/1 -> T4/1
  PWM1/1 -> NOT/1, T1/1

== system FOC_physical_2/SVPWM Technique/PWM ==
  Ts1 : Inport
  Ts3 : Inport  Port=2
  Ts5 : Inport  Port=3
  Carrier : Inport  Port=4
  Mux : Mux  Inputs=2
  Relational Operator : RelationalOperator  OutDataTypeStr=boolean  RndMeth=Simplest  InputSameDT=off
  Relational Operator1 : RelationalOperator  OutDataTypeStr=boolean  RndMeth=Simplest  InputSameDT=off
  Relational Operator2 : RelationalOperator  OutDataTypeStr=boolean  RndMeth=Simplest  InputSameDT=off
  Scope : Scope  NumInputPorts=2
  PWM1 : Outport
  PWM3 : Outport  Port=2
  PWM5 : Outport  Port=3
  wires:
  Mux/1 -> Scope/1
  Relational Operator2/1 -> PWM5/1
  Relational Operator1/1 -> PWM3/1
  Relational Operator/1 -> PWM1/1, Scope/2
  Carrier/1 -> Relational Operator/2, Mux/2, Relational Operator1/2, Relational Operator2/2
  Ts5/1 -> Relational Operator2/1
  Ts3/1 -> Relational Operator1/1
  Ts1/1 -> Relational Operator/1, Mux/1

== system FOC_physical_2/SVPWM Technique/Step 1- Determine Vd, Vq, Vref, and angle ==
  Va* : Inport
  Vb* : Inport  Port=2
  Vc* : Inport  Port=3
  Polar form : Subsystem
  "Power variant Clark transformation " : Subsystem
  Scope : Scope  NumInputPorts=2
  V ref : Outport
  angle : Outport  Port=2
  wires:
  Vc*/1 -> "Power variant Clark transformation "/3(Vc)
  Vb*/1 -> "Power variant Clark transformation "/2(Vb)
  Va*/1 -> "Power variant Clark transformation "/1(Va)
  Polar form/2(angle) -> angle/1
  Polar form/1(V ref) -> V ref/1
  "Power variant Clark transformation "/2(V beta) -> Polar form/2(In2), Scope/2
  "Power variant Clark transformation "/1(V alpha) -> Polar form/1(In1), Scope/1

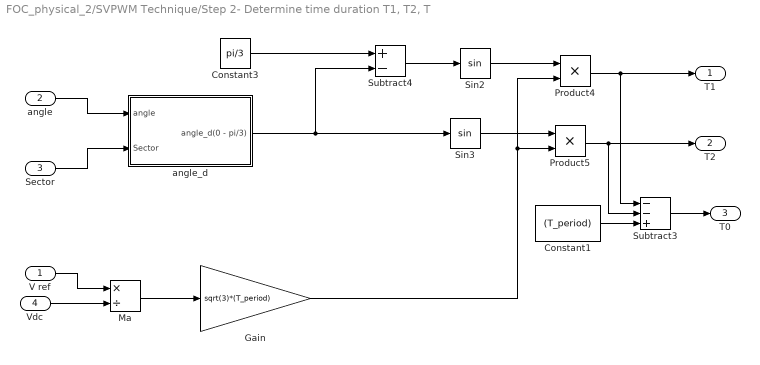
== system FOC_physical_2/SVPWM Technique/Step 2- Determine time duration T1, T2, T ==
  V ref : Inport
  angle : Inport  Port=2
  Sector : Inport  Port=3
  Vdc : Inport  Port=4
  Constant1 : Constant  Value=(T_period)
  Constant3 : Constant  Value=pi/3
  Gain : Gain  Gain=sqrt(3)*(T_period)
  Ma : Product  Inputs=*/
  Product4 : Product
  Product5 : Product
  Sin2 : Trigonometry
  Sin3 : Trigonometry
  Subtract3 : Sum  Inputs=--+
  Subtract4 : Sum  Inputs=+-
  angle_d : Subsystem
  T1 : Outport
  T2 : Outport  Port=2
  T0 : Outport  Port=3
  wires:
  angle_d/1(angle_d(0 - pi/3)) -> Subtract4/2, Sin3/1
  Constant1/1 -> Subtract3/3
  Subtract3/1 -> T0/1
  Product5/1 -> T2/1, Subtract3/2
  Sin3/1 -> Product5/1
  Product4/1 -> T1/1, Subtract3/1
  Gain/1 -> Product5/2, Product4/2
  Sin2/1 -> Product4/1
  Ma/1 -> Gain/1
  Subtract4/1 -> Sin2/1
  Constant3/1 -> Subtract4/1
  Vdc/1 -> Ma/2
  V ref/1 -> Ma/1
  Sector/1 -> angle_d/2(Sector)
  angle/1 -> angle_d/1(angle)

== system FOC_physical_2/SVPWM Technique/Step 3- Determine the switching time of each transistor (S1 to S6)  ==
  T1 : Inport
  T2 : Inport  Port=2
  T0 : Inport  Port=3
  S : Inport  Port=4
  Fcn : Fcn  Expr=(T_period)-u(3)/2
  Fcn1 : Fcn  Expr=u(3)/2+u(2)
  Fcn2 : Fcn  Expr=u(3)/2
  Fcn3 : Fcn  Expr=u(3)/2+u(1)
  Mux1 : Mux  Inputs=3
  Sector detection1 : MATLAB Function  TreatAsAtomicUnit=on
  Ts1 : Outport
  Ts3 : Outport  Port=2
  Ts5 : Outport  Port=3
  wires:
  Sector detection1/1(Ts1) -> Ts1/1
  Sector detection1/3(Ts5) -> Ts5/1
  Sector detection1/2(Ts3) -> Ts3/1
  T0/1 -> Mux1/3
  T2/1 -> Mux1/2
  T1/1 -> Mux1/1
  Fcn2/1 -> Sector detection1/4(w)
  Fcn/1 -> Sector detection1/2(u)
  Fcn3/1 -> Sector detection1/5(g)
  Mux1/1 -> Fcn2/1, Fcn3/1, Fcn1/1, Fcn/1
  Fcn1/1 -> Sector detection1/3(v)
  S/1 -> Sector detection1/1(s)

== system FOC_physical_2/Subsystem/Forward Clacke ==
  Iu : Inport
  Iv : Inport  Port=2
  Iw : Inport  Port=3
  Gain : Gain  Gain=0.5
  Gain1 : Gain  Gain=0.5
  Gain2 : Gain  Gain=2/3
  Gain3 : Gain  Gain=sqrt(3)/2
  Gain4 : Gain  Gain=2/3
  Sum : Sum  Inputs=+--
  Sum1 : Sum  Inputs=+-
  I_alpha : Outport
  I_beta : Outport  Port=2
  wires:
  Iv/1 -> Gain/1, Sum1/1
  Gain/1 -> Sum/2
  Gain2/1 -> I_alpha/1
  Sum1/1 -> Gain3/1
  Gain1/1 -> Sum/3
  Iw/1 -> Gain1/1, Sum1/2
  Sum/1 -> Gain2/1
  Gain3/1 -> Gain4/1
  Iu/1 -> Sum/1
  Gain4/1 -> I_beta/1

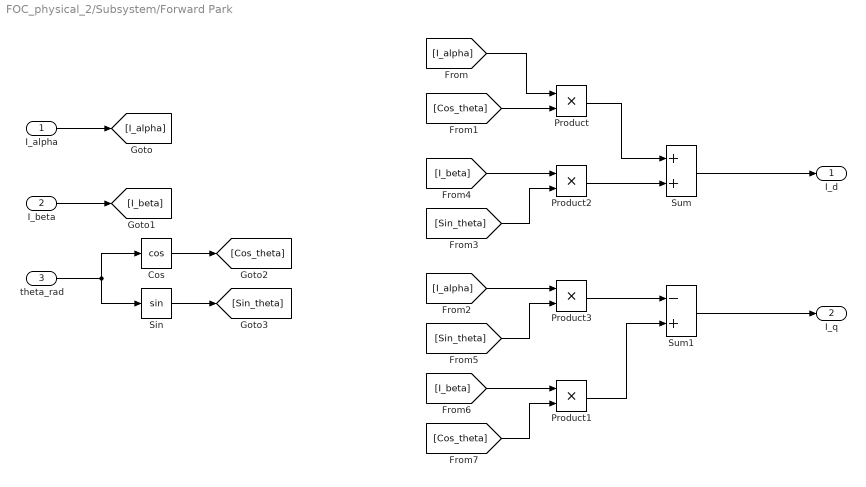
== system FOC_physical_2/Subsystem/Forward Park ==
  I_alpha : Inport
  I_beta : Inport  Port=2
  theta_rad : Inport  Port=3
  Cos : Trigonometry  Operator=cos
  Product{,1..3} (4 alike) : Product
  Sin : Trigonometry
  Sum : Sum
  Sum1 : Sum  Inputs=-+
  I_d : Outport
  I_q : Outport  Port=2
  wires:
  [Cos_theta] -> Product1/2
  [I_beta] -> Product1/1
  [Sin_theta] -> Product3/2
  [I_alpha] -> Product3/1
  Product1/1 -> Sum1/2
  [I_beta] -> Product2/1
  [Sin_theta] -> Product2/2
  [Cos_theta] -> Product/2
  Sin/1 -> [Sin_theta]
  Cos/1 -> [Cos_theta]
  theta_rad/1 -> Cos/1, Sin/1
  [I_alpha] -> Product/1
  I_beta/1 -> [I_beta]
  I_alpha/1 -> [I_alpha]
  Product3/1 -> Sum1/1
  Product2/1 -> Sum/2
  Product/1 -> Sum/1
  Sum1/1 -> I_q/1
  Sum/1 -> I_d/1

== system FOC_physical_2/Subsystem/Inverse Transformation ==
  Vq : Inport
  theta : Inport  Port=2
  Vd : Inport  Port=3
  "Inverse Park " : Subsystem  Commented=on
  dq to abc : Subsystem
  inverse Clark : Subsystem  Commented=on
  Va : Outport
  Vb : Outport  Port=2
  Vc : Outport  Port=3
  wires:
  theta/1 -> dq to abc/3(theta)
  Vq/1 -> dq to abc/1(V_q*)
  Vd/1 -> dq to abc/2(V_d*)
  dq to abc/1(Va*) -> Va/1
  dq to abc/2(Vb*) -> Vb/1
  dq to abc/3(Vc*) -> Vc/1

== system FOC_physical_2/Subsystem/SPWM BLOCK ==
  Va : Inport
  Vb : Inport  Port=2
  Vc : Inport  Port=3
  V_DC : Inport  Port=4
  Out1 : Outport
  wires:
  Va/1 -> Out1/1

== system FOC_physical_2/Subsystem/SVPWM1 ==
  Va : Inport
  Vb : Inport  Port=2
  Vc : Inport  Port=3
  Vdc : Inport  Port=4
  Scope : Scope  NumInputPorts=3
  Scope4 : Scope  NumInputPorts=4
  Sector detection : MATLAB Function  TreatAsAtomicUnit=on
  Subsystem : Subsystem
  Subsystem1 : Subsystem
  Subsystem2 : Subsystem
  Subsystem3 : Subsystem  Commented=on
  Subsystem4 : Subsystem  Commented=on
  Valpha and Vbeta Clark Trans : Subsystem
  TS1 : Outport
  TS3 : Outport  Port=2
  TS5 : Outport  Port=3
  wires:
  Vdc/1 -> Subsystem1/4(Vdc)
  Subsystem2/3(TS5) -> TS5/1
  Subsystem2/1(TS1) -> TS1/1
  Subsystem2/2(TS3) -> TS3/1
  Subsystem1/3(T0) -> Scope4/3, Subsystem2/3(T0)
  Subsystem1/1(T1) -> Subsystem2/1(T1), Scope4/1
  Subsystem1/2(T2) -> Subsystem2/2(T2), Scope4/2
  Sector detection/1(S) -> Subsystem2/4(Sector definiton), Subsystem1/3(Sector)  "Sector definiton"
  Subsystem/1(Vref) -> Subsystem1/1(Vref)
  Va/1 -> Scope/1, Valpha and Vbeta Clark Trans/1(Va)
  Vc/1 -> Valpha and Vbeta Clark Trans/3(Vc), Scope/3
  Subsystem/2(angle) -> Subsystem1/2(angle), Sector detection/1(u)
  Vb/1 -> Valpha and Vbeta Clark Trans/2(Vb), Scope/2
  Valpha and Vbeta Clark Trans/2(Vbeta) -> Subsystem/2(Vbeta)
  Valpha and Vbeta Clark Trans/1(Valpha) -> Subsystem/1(Valpha)
